simulink model "FAS_Kreuzungswarner_Simulation_V1"  (R2024b)
settings: Solver=FixedStepAuto  StartTime=0.0  StopTime=stoptime  FixedStep=sampletime  RelTol=1e-3
InitFcn:
  | if ~evalin('base', 'exist(''Auswertungsflag'', ''var'')') || evalin('base', 'Auswertungsflag.Value == 0')
  |     Parameterskript;
  |     run('StartGUI');  % explizit ausführen (nicht blockierend!)
  | end
values from neighbouring files (symbols this model uses):
  mEGO = str2double(massEGOInput.String)    [StartGUI.m]
  mFZG = str2double(massFZGInput.String)    [StartGUI.m]
  OeffnungswinkelA = str2double(angleInputA.String)    [StartGUI.m]
  OeffnungswinkelB = Simulink.Parameter    [Auswertung.m]    (also in StartGUI.m = str2double(angleInputB.String))
  P_EGO = str2double(powerEGOInput.String)    [StartGUI.m]
  P_FZG = str2double(powerFZGInput.String)    [StartGUI.m]
  ReichweiteA = str2double(rangeInputA.String)    [StartGUI.m]
  ReichweiteB = str2double(rangeInputB.String)    [StartGUI.m]
  SensorA = sensor1Dropdown.Value    [StartGUI.m]
  SensorB = sensor2Dropdown.Value    [StartGUI.m]
  startPositionEGO = str2double(posEGOInput.String)    [StartGUI.m]
  startPositionFzg = str2double(posFzgInput.String)    [StartGUI.m]
  v_EGO = str2double(velEGOInput.String)    [StartGUI.m]
  v_FZG = str2double(velFZGInput.String)    [StartGUI.m]
  Wetter = weatherDropdown.Value    [StartGUI.m]
  zweitesFzgSwitch = str2double(zweitesFzgInput.String)    [StartGUI.m]
undefined symbols (not defined in the file or in its folder): Airbagzeit, Ausloesezeit, b, dt, g, Haltezeit, l, munass, muschnee, mutrocken, rad_b, rad_l, reifen_dx, reifen_dy, SensorSwitch, startPositionFzg2, xFZG, yEGO
(part 3 of 3)

== matlab function FAS_Kreuzungswarner_Simulation_V1/Visualisierung/OneCar - World View ==
  settings: updateMethod=DISCRETE
  data: xEGO input; xFzg2 input; Passive_Sicherheit input; Bremswarnung input; warningHMI input; yFZG input; yEGO parameter; xFZG parameter; b parameter; l parameter; rad_b parameter; rad_l parameter; reifen_dx parameter; reifen_dy parameter; OeffnungswinkelB parameter; ReichweiteB parameter; ReichweiteA parameter size=1; OeffnungswinkelA parameter size=1; startPositionFzg2 parameter size=1; Wetter parameter size=1; SensorSwitch parameter size=1; SensorB parameter size=1; zweitesFzgSwitch parameter size=1
%% Allgemeine Informationen ===================================================================================
% Visualisierung eines EGO-Fahrzeugs und eines weiteren Fahrzeugs in einer 2D-Umgebung.
% - Zusatzmöglichkeit mit vorrausfahrendem Fahrzeug
% Ziel: Darstellung der Fahrzeugsimulation, Reifen, Stoßstangen und zweier Sensorkegel (grün und gelb).

% Sensorumschaltung: Umschalten von Öffnungswinkel und Reichweite mit Farbunterschied 
% - Umschalten geschieht im Parameterskript
% - Switch.Value = 0: Zeige nur gelben Kegel (B) mit kleiner Reichweite und Öffnungswinkel
% - Switch.Value = 1: Zeige grünen Kegel (A) mit großer Reichweite + gelben Kegel (B)

% Ausgabe erfolgt in zwei Figure:
% - Figure 1: Fahrzeugwelt
% - Figure 2: HMI-Warnmeldungen (Bremsung, Abstand, Passive Sicherheit)

% Variablen aus Parameter oder Input erkennen
% - Variablen welche aus dem Parameterskript kommen können über -> Function -> Edit Data bearbeitet werden 
% - Variablen welche als Input verwendet werden haben einen Port zugewiesen

% Debuggen: Wertausgabe im Diagnosefenster
% - disp("Variable");
% ===============================================================================================================

%% Beschreibung der Funktionsargumente welche die Funktion übergeben kriegt =====================================
% - xEGO und yFZG: Startpositionen
% - yEGO und xFZG: der Offset auf die Spurmitte
% - b und l: Breite und Länge der Autos
% - rad_b und rad_l: Breite und Länge der Reifen
% - reifen_dx und reifen_dy: offset der Reifen ins Fahrzeuginnere
% - Oeffnungswinkel und Reichweite: Sensorkegelgröße
% - Regen: Switch ob Aktiv (in GUI auswählen)
% - SensorSwitch: Umschalten geschieht im Parameterskript 0/1 hinzufügen von komplettem Erfassen
% - SensorB: auswahl in GUI ob Radar, Kamera oder kein Kegel (---)
% - zweitesFzgSwitch: aktivieren in GUI mit letztem Szenario (vorrausfahrendes Fahrzeug)
% - startPositionFzg2: offset zum EGO
% ===============================================================================================================

%% Initialisierung und Aktualisierung ===========================================================================
% - Initialisierung der Figur und der Fahrzeuggrafik erfolgt nur einmal (bei erstem Aufruf).
% - Der Zustand der Fahrzeuge und Sensorkegel wird dann in jedem Simulationsschritt aktualisiert.
% - Das zweite Fahrzeug wird nur gezeichnet und aktualisiert, wenn zweitesFzgSwitch == 1.
% - Kegel (Sensorkegel) werden einmal erstellt und bei jedem Schritt basierend auf Position und 
%   SensorSwitch aktualisiert.
% - Die HMI-Meldungen (Bremswarnung, Passive Sicherheit, Regen) werden in einer separaten Figure angezeigt.
% ===============================================================================================================


%% Hauptfunktion ==================================================================================================================================================================================

function Visualisierung(xEGO, xFzg2, Passive_Sicherheit, Bremswarnung, warningHMI, yFZG, ...   % Port Input 
                        yEGO, xFZG, b, l, rad_b, rad_l, reifen_dx, reifen_dy,OeffnungswinkelB, ReichweiteB, ReichweiteA, OeffnungswinkelA, startPositionFzg2, ... % Parameterskript Variablen fest
                        Wetter, SensorSwitch, SensorB, zweitesFzgSwitch) % Parameterskript Switch über GUI variabel
    

    %% Persistent-Variablen (nur beim ersten Aufruf initialisieren)
    persistent PosEGO PosFZG PosEGO_Bumper PosFZG_Bumper     
    persistent EGO_R1 EGO_R2 EGO_R3 EGO_R4  % R = Reifen (Radkasten)
    persistent FZG_R1 FZG_R2 FZG_R3 FZG_R4
    persistent PosFZG2 PosFZG2_Bumper FZG2_R1 FZG2_R2 FZG2_R3 FZG2_R4
    persistent kegel_gruen kegel_gelb
    
    %% Sicherstellen, dass beide Figures existieren
    fig1 = findobj('Type', 'figure', 'Number', 1);
    if isempty(fig1)
        figure(1);
        init_figure_world();
    end
    
    fig2 = findobj('Type', 'figure', 'Number', 2);
    if isempty(fig2)
        figure(2);
        clf; hold on; axis equal;
        axis([-30 30 -30 30]);
        title('HMI Meldungen');
    end

   
    %% Initialisierungen bei erstem Aufruf

    if isempty(PosEGO)          % Nur einmal Plot Initialisieren
        
        % Erstellen der Figure (Funktionsaufruf)
        init_figure_world();
        
        % Initialisieren der Kegel
        if isempty(kegel_gruen)
            kegel_gruen = init_sensorkegel(xEGO, yEGO, l, OeffnungswinkelA, ReichweiteA, SensorB, 'g');
        end
        if isempty(kegel_gelb)
            kegel_gelb = init_sensorkegel(xEGO, yEGO, l, OeffnungswinkelB, ReichweiteB, SensorB, 'y');
        end
        
        % Initialisierung Fahrzeuge (Funktionsaufruf)
        [PosEGO, PosFZG, PosEGO_Bumper, PosFZG_Bumper, ...
        EGO_R1, EGO_R2, EGO_R3, EGO_R4, ...
        FZG_R1, FZG_R2, FZG_R3, FZG_R4, ...
        l, b, rad_b, rad_l, reifen_dx, reifen_dy] = ...
        init_plot_fahrzeug(xEGO, yFZG, yEGO, xFZG, l, b, rad_b, rad_l, reifen_dx, reifen_dy);

        % Zweites Fahrzeug initialisieren, falls Switch aktiv ist
        if zweitesFzgSwitch == 1
            [PosFZG2, PosFZG2_Bumper, FZG2_R1, FZG2_R2, FZG2_R3, FZG2_R4] = ...
                init_zweites_fzg(xEGO + startPositionFzg2, yEGO, l, b, rad_b, rad_l, reifen_dx, reifen_dy);
        else
            % Leere Variablen für das zweite Fahrzeug (sind aber definiert)
            PosFZG2 = [];
            PosFZG2_Bumper = [];
            FZG2_R1 = []; FZG2_R2 = []; FZG2_R3 = []; FZG2_R4 = [];
        end
        
    end
    
    %% Aktualisierung der Visualisierung
    
    % Aktualisierung Fahrzeug (Funktionsaufruf)
    update_plot_fahrzeug(xEGO, yEGO, xFZG, yFZG, ...
                        PosEGO, PosFZG, ...
                        PosEGO_Bumper, PosFZG_Bumper, ...
                        EGO_R1, EGO_R2, EGO_R3, EGO_R4, ...
                        FZG_R1, FZG_R2, FZG_R3, FZG_R4, ...
                        l, b, rad_l, rad_b, reifen_dx, reifen_dy);

    % Zweites Fahrzeug aktualisieren falls vorhanden
    if zweitesFzgSwitch == 1
        update_zweites_fzg(PosFZG2, PosFZG2_Bumper, FZG2_R1, FZG2_R2, FZG2_R3, FZG2_R4, ...
                           xFzg2 + startPositionFzg2, yEGO, l, b, rad_b, rad_l, reifen_dx, reifen_dy);
    end
        
    % Sensorkegel aktualisieren und Sichtbarkeit setzen 
    if isempty(kegel_gelb)
        kegel_gruen = init_sensorkegel(xEGO, yEGO, l, OeffnungswinkelA, ReichweiteA, SensorB, 'g');
    end
    if isempty(kegel_gelb)
        kegel_gelb = init_sensorkegel(xEGO, yEGO, l, OeffnungswinkelB, ReichweiteB, SensorB, 'y');
    end
    
    update_sensorkegel(kegel_gruen, l, xEGO, yEGO, OeffnungswinkelA, ReichweiteA, SensorB);
    update_sensorkegel(kegel_gelb,  l, xEGO, yEGO, OeffnungswinkelB, ReichweiteB, SensorB);
    
    % Sichtbarkeit je nach Modus setzen
    if SensorSwitch == 0
        set(kegel_gruen, 'Visible', 'off');
        set(kegel_gelb,  'Visible', 'on');
    else
        set(kegel_gruen, 'Visible', 'on');
        set(kegel_gelb,  'Visible', 'on');
    end
    
    % warningHMI, Bremswarnung, Passive Sicherheit (Funktionsaufruf)
    aktor_warnungen(Bremswarnung, Passive_Sicherheit, warningHMI, Wetter);
      
    % Aktualisieren der Darstellung
    drawnow;

end



%% == Funktionen =========================================================================================


%% == Initialisierung der Figure (Hintergrund und Straßenmarkierungen) ==============================
function init_figure_world()

    % Neue Figur mit bestimmter Position
    figure(1);
    clf;  % Figur leeren, falls sie schon existierte
    hold on; grid on; axis equal;
    axis([-50 50 -50 50]);

    xlabel('X-Position'); ylabel('Y-Position');
    title('Fahrzeugbewegung');

    % Hintergrund
    fill([-50 50 50 -50], [-50 -50 50 50], [0 1 0]*0.8, 'Edgecolor', 'none');
    fill([-50 50 50 -50], [-5 -5 5 5], [1 1 1]*0.7, 'Edgecolor', 'none');
    fill([-5 -5 5 5], [-50 50 50 -50], [1 1 1]*0.7, 'Edgecolor', 'none');

    % Straßenmarkierungen
    plot([-50 -5], [-5 -5], 'w', 'LineWidth', 2);
    plot([5 50], [-5 -5], 'w', 'LineWidth', 2);
    plot([-50 -5], [5 5], 'w', 'LineWidth', 2);
    plot([5 50], [5 5], 'w', 'LineWidth', 2);
    plot([-5 -5], [50 5], 'w', 'LineWidth', 2);
    plot([5 5], [50 5], 'w', 'LineWidth', 2);
    plot([-5 -5], [-5 -50], 'w', 'LineWidth', 2);
    plot([5 5], [-5 -50], 'w', 'LineWidth', 2);

    % Fahrbahnmarkierungen
    plot([-50 -5], [0 0], 'w--', 'LineWidth', 2);
    plot([5 50], [0 0], 'w--', 'LineWidth', 2);
    plot([0 0], [50 5], 'w--', 'LineWidth', 2);
    plot([0 0], [-5 -50], 'w--', 'LineWidth', 2);

end

%% Initialisierung (Fahrzeuge, Stoßstange, Funktionsaufruf Reifen)
function [PosEGO, PosFZG, PosEGO_Bumper, PosFZG_Bumper, ...
          EGO_R1, EGO_R2, EGO_R3, EGO_R4, ...
          FZG_R1, FZG_R2, FZG_R3, FZG_R4, ...
          l, b, rad_b, rad_l, reifen_dx, reifen_dy] = ...
          init_plot_fahrzeug(xEGO, yFZG, yEGO, xFZG, l, b, rad_b, rad_l, reifen_dx, reifen_dy)

    % Fahrzeugkörper EGO zeichnen
    PosEGO = fill([xEGO-l/2 xEGO+l/2 xEGO+l/2 xEGO-l/2], ...
                  [yEGO-b/2 yEGO-b/2 yEGO+b/2 yEGO+b/2], 'b');
    % Stoßstangen EGO
    PosEGO_Bumper = plot([xEGO+l/2 xEGO+l/2], [yEGO+b/2 yEGO-b/2], 'k-', 'LineWidth', 2.5);
    % Räder zeichnen
    [EGO_R1, EGO_R2, EGO_R3, EGO_R4] = plot_raeder(xEGO, yEGO, l, b, rad_l, rad_b, reifen_dx, reifen_dy, 'k');

    % Fahrzeugkörper FZG zeichnen
    PosFZG = fill([xFZG-b/2 xFZG+b/2 xFZG+b/2 xFZG-b/2], ...
                  [yFZG-l/2 yFZG-l/2 yFZG+l/2 yFZG+l/2], 'g');
    % Stoßstangen FZG
    PosFZG_Bumper = plot([xFZG-b/2 xFZG+b/2], [yFZG+l/2 yFZG+l/2], 'k-', 'LineWidth', 2.5);
    % Räder zeichnen
    [FZG_R1, FZG_R2, FZG_R3, FZG_R4] = plot_raeder(xFZG, yFZG, b, l, rad_b, rad_l, reifen_dx, reifen_dy, 'k');

end

%% Aktualisiert Fahrzeuge, Stoßstange, Funktionsaufruf Reifen (bei jedem Schritt)
function update_plot_fahrzeug(xEGO, yEGO, xFZG, yFZG, ...
                             PosEGO, PosFZG, ...
                             PosEGO_Bumper, PosFZG_Bumper, ...
                             EGO_R1, EGO_R2, EGO_R3, EGO_R4, ...
                             FZG_R1, FZG_R2, FZG_R3, FZG_R4, ...
                             l, b, rad_l, rad_b, reifen_dx, reifen_dy)

    % EGO Fahrzeugkörper aktualisieren
    set(PosEGO, 'XData', [xEGO-l/2 xEGO+l/2 xEGO+l/2 xEGO-l/2]);
    set(PosEGO, 'YData', [yEGO-b/2 yEGO-b/2 yEGO+b/2 yEGO+b/2]);

    % EGO Stoßstange aktualisieren
    set(PosEGO_Bumper, 'XData', [xEGO+l/2 xEGO+l/2]);
    set(PosEGO_Bumper, 'YData', [yEGO+b/2 yEGO-b/2]);

    % FZG Fahrzeugkörper aktualisieren
    set(PosFZG, 'XData', [xFZG-b/2 xFZG+b/2 xFZG+b/2 xFZG-b/2]);
    set(PosFZG, 'YData', [yFZG-l/2 yFZG-l/2 yFZG+l/2 yFZG+l/2]);

    % FZG Stoßstange aktualisieren
    set(PosFZG_Bumper, 'XData', [xFZG-b/2 xFZG+b/2]);
    set(PosFZG_Bumper, 'YData', [yFZG+l/2 yFZG+l/2]);

    % Räder EGO updaten Funktion
    update_raeder(EGO_R1, EGO_R2, EGO_R3, EGO_R4, ...
                  xEGO, yEGO, l, b, rad_l, rad_b, reifen_dx, reifen_dy);
    
    % Räder FZG updaten Funktion
    update_raeder(FZG_R1, FZG_R2, FZG_R3, FZG_R4, ...
                  xFZG, yFZG, b, l, rad_b, rad_l, reifen_dx, reifen_dy);

end

%% Initialisierung (zweites Fahrzeug, Stoßstange, Funktionsaufruf Reifen) falls switch aktiv
function [PosFZG2, PosFZG2_Bumper, FZG2_R1, FZG2_R2, FZG2_R3, FZG2_R4] = ...
          init_zweites_fzg(x, y, l, b, rad_b, rad_l, reifen_dx, reifen_dy)
      
    % Fahrzeugkörper zeichnen
    PosFZG2 = fill([x - l/2, x + l/2, x + l/2, x - l/2], ...
                   [y - b/2, y - b/2, y + b/2, y + b/2], 'r');  % Rot für zweites Fahrzeug
    
    % Stoßstange
    PosFZG2_Bumper = plot([x + l/2, x + l/2], [y + b/2, y - b/2], 'k-', 'LineWidth', 2.5);
    
    % Räder zeichnen
    [FZG2_R1, FZG2_R2, FZG2_R3, FZG2_R4] = plot_raeder(x, y, l, b, rad_l, rad_b, reifen_dx, reifen_dy, 'k');

end

%% Aktualisiert zweites Fahrzeug, Stoßstange, Funktionsaufruf Reifen (bei jedem Schritt)
function update_zweites_fzg(PosFZG2, PosFZG2_Bumper, FZG2_R1, FZG2_R2, FZG2_R3, FZG2_R4, ...
                            x, y, l, b, rad_b, rad_l, reifen_dx, reifen_dy)
    
    % Fahrzeugkörper aktualisieren
    set(PosFZG2, 'XData', [x - l/2, x + l/2, x + l/2, x - l/2]);
    set(PosFZG2, 'YData', [y - b/2, y - b/2, y + b/2, y + b/2]);
    
    % Stoßstange aktualisieren
    set(PosFZG2_Bumper, 'XData', [x + l/2, x + l/2]);
    set(PosFZG2_Bumper, 'YData', [y + b/2, y - b/2]);
    
    % Räder aktualisieren
    update_raeder(FZG2_R1, FZG2_R2, FZG2_R3, FZG2_R4, ...
                  x, y, l, b, rad_l, rad_b, reifen_dx, reifen_dy);

end

%% Initialisiert die Räder (einmalig)  
function [reifen_HL, reifen_HR, reifen_VR, reifen_VL] = ...
    plot_raeder(x, y, l, b, rad_l, rad_b, reifen_dx, reifen_dy, color)
    
    % 4x2 Matrix (Äußere Reifenecke) mit Bezug auf EGO in X-Richtung ->
    pos = [
            -l/2 + reifen_dx, -b/2 + reifen_dy; 
            -l/2 + reifen_dx,  b/2 - reifen_dy;
             l/2 - reifen_dx, -b/2 + reifen_dy;   
             l/2 - reifen_dx,  b/2 - reifen_dy
          ];

    reifen_HL = fill([x+pos(1,1), x+pos(1,1)+rad_l, x+pos(1,1)+rad_l, x+pos(1,1)], ... 
                [y+pos(1,2), y+pos(1,2), y+pos(1,2)+rad_b, y+pos(1,2)+rad_b], color);
    reifen_HR = fill([x+pos(2,1), x+pos(2,1)+rad_l, x+pos(2,1)+rad_l, x+pos(2,1)], ...
                [y+pos(2,2), y+pos(2,2), y+pos(2,2)-rad_b, y+pos(2,2)-rad_b], color);
    reifen_VR = fill([x+pos(3,1), x+pos(3,1), x+pos(3,1)-rad_l, x+pos(3,1)-rad_l], ...
                [y+pos(3,2), y+pos(3,2)+rad_b, y+pos(3,2)+rad_b, y+pos(3,2)], color);
    reifen_VL = fill([x+pos(4,1), x+pos(4,1), x+pos(4,1)-rad_l, x+pos(4,1)-rad_l], ...
                [y+pos(4,2), y+pos(4,2)-rad_b, y+pos(4,2)-rad_b, y+pos(4,2)], color);

end

%% Aktualisiert die Räder (bei jedem Schritt)
function update_raeder(reifen_HL, reifen_HR, reifen_VR, reifen_VL, x, y, l, b, rad_l, rad_b, reifen_dx, reifen_dy)
    
    % 4x2 Matrix (Äußere Reifenecke) mit Bezug auf EGO in X-Richtung ->
    pos = [
            -l/2 + reifen_dx, -b/2 + reifen_dy; 
            -l/2 + reifen_dx,  b/2 - reifen_dy;
             l/2 - reifen_dx, -b/2 + reifen_dy;   
             l/2 - reifen_dx,  b/2 - reifen_dy
          ];

    set(reifen_HL, 'XData', [x+pos(1,1), x+pos(1,1)+rad_l, x+pos(1,1)+rad_l, x+pos(1,1)], ...
                   'YData', [y+pos(1,2), y+pos(1,2), y+pos(1,2)+rad_b, y+pos(1,2)+rad_b]);
    set(reifen_HR, 'XData', [x+pos(2,1), x+pos(2,1)+rad_l, x+pos(2,1)+rad_l, x+pos(2,1)], ...
                   'YData', [y+pos(2,2), y+pos(2,2), y+pos(2,2)-rad_b, y+pos(2,2)-rad_b]);
    set(reifen_VR, 'XData', [x+pos(3,1), x+pos(3,1), x+pos(3,1)-rad_l, x+pos(3,1)-rad_l], ...
                   'YData', [y+pos(3,2), y+pos(3,2)+rad_b, y+pos(3,2)+rad_b, y+pos(3,2)]);
    set(reifen_VL, 'XData', [x+pos(4,1), x+pos(4,1), x+pos(4,1)-rad_l, x+pos(4,1)-rad_l], ...
                   'YData', [y+pos(4,2), y+pos(4,2)-rad_b, y+pos(4,2)-rad_b, y+pos(4,2)]);

end

%% Aktor Warnungen Plot (HMI, Bremswarnung, Passive Sicherheit, Regen)
function aktor_warnungen(Bremswarnung, Passive_Sicherheit, warningHMI, Regen)
    
    % Figure 2 für HMI
    figure(2); clf;  % ID für einmaligen Aufruf
    hold on; axis equal;
    axis([-30 30 -30 30]);

    % Beschriftung
    title('HMI Meldungen');

    % HMI Meldung
    if warningHMI == 1
       fill([-25 25 25 -25], [17.5 17.5 27.5 27.5], [1 1 1]*1);
       text(-17, 22.5,'Warnung Abstand','color','red', 'FontWeight','bold', 'FontSize', 16)
    end 
    
    % Warnung Bremsen
    if Bremswarnung == 1
       fill([-25 25 25 -25], [2.5 2.5 12.5 12.5], [1 1 1]*1);
       text(-17, 7.5,'Warnung Bremsen','color','red', 'FontWeight','bold', 'FontSize', 16)
    end

    % Aktivierung der Passiven Sicherheit
    if Passive_Sicherheit == 1
       fill([-25 25 25 -25], [-12.5 -12.5 -2.5 -2.5], [1 1 1]*1);
       text(-17, -7.5,'Passive Sicherheit','color','red', 'FontWeight','bold', 'FontSize', 16)
    end 
    
    % Regenwarnung
    if Regen == 2
        fill([-25 25 25 -25], [-27.5 -27.5 -17.5 -17.5], [1 1 1]*1);
        text(-11, -22.5,'Regen Aktiv','color','blue', 'FontWeight','bold', 'FontSize', 16)
    end

    % Schneewarnung
    if Regen == 3
        fill([-25 25 25 -25], [-27.5 -27.5 -17.5 -17.5], [1 1 1]*1);
        text(-11, -22.5,'Schnee Aktiv','color','blue', 'FontWeight','bold', 'FontSize', 16)
    end

end

%% Initialisiert den Sensorkegel (einmalig)
function kegel_sensor = init_sensorkegel(xEGO, yEGO, l, Oeffnungswinkelx, Reichweitex, SensorB, color)
    
    % Kein Kegel anzeigen
    if SensorB == 3
        Oeffnungswinkelx = 0;
        Reichweitex = 0;
    end

    anzahl_punkte = 100;

    x0 = xEGO + l/2;
    y0 = yEGO;

    winkel_vec = linspace(-Oeffnungswinkelx/2, Oeffnungswinkelx/2, anzahl_punkte);
    x_bogen = x0 + Reichweitex * cosd(winkel_vec);
    y_bogen = y0 + Reichweitex * sind(winkel_vec);

    x_fill = [x0, x_bogen, x0];
    y_fill = [y0, y_bogen, y0];

    kegel_sensor = fill(x_fill, y_fill, color, 'FaceAlpha', 0.4, 'EdgeColor', 'none');

end

%% Aktualisiert den Sensorkegel (bei jedem Schritt)
function update_sensorkegel(kegel_sensor, l, xEGO, yEGO, Oeffnungswinkelx, Reichweitex, SensorB)

    % Kein Kegel anzeigen
    if SensorB == 3
        Oeffnungswinkelx = 0;
        Reichweitex = 0;
    end
    anzahl_punkte = 100;

    x0 = xEGO + l/2;
    y0 = yEGO;

    winkel_vec = linspace(-Oeffnungswinkelx/2, Oeffnungswinkelx/2, anzahl_punkte);
    x_bogen = x0 + Reichweitex * cosd(winkel_vec);
    y_bogen = y0 + Reichweitex * sind(winkel_vec);

    x_fill = [x0, x_bogen, x0];
    y_fill = [y0, y_bogen, y0];

    set(kegel_sensor, 'XData', x_fill, 'YData', y_fill);
    
end
